simulink model "s_FPID_SOPDTUZ"  (R2022a)
settings: Solver=ode45  StartTime=0.0  StopTime=simT  MaxStep=Tsm  RelTol=rtol  AbsTol=atol
values from neighbouring files (symbols this model uses):
  beta = c0(5)+c1(5)*a+c2(5)*b+c3(5)*a*b+c4(5)*b^2+c5(5)*a*b^2+c6(5)*b^3    [PID_MoReRT.m]
  D1 = [T^2 2*T 1]    [Figure_08.m]    (also in PD1nR_2DOF_Qn.m; PD3nR_2DOF_Qn.m; PD5nR_2DOF_Qn.m; PD7nR_2DOF_Qn.m)
  di0 = 0    [Figure_03a_above.m]    (also in Figure_03b_middle.m; Figure_03c_below.m; Figure_04.m; Figure_05.m)
  di1 = 1    [Figure_03a_above.m]    (also in Figure_03b_middle.m; Figure_03c_below.m; Figure_04.m; Figure_05.m)
  do = 0    [Figure_03a_above.m]    (also in Figure_03b_middle.m; Figure_03c_below.m; Figure_04.m; Figure_05.m)
  do0 = 0    [Figure_03a_above.m]    (also in Figure_03b_middle.m; Figure_03c_below.m; Figure_04.m; Figure_05.m)
  dy = .1    (= 0.1)    [Figure_03a_above.m]    (also in Figure_03b_middle.m; Figure_03c_below.m; Figure_04.m = 0.05; Figure_05.m = 0.05)
  Kdy = 0    [Figure_03a_above.m]    (also in Figure_03b_middle.m; Figure_03c_below.m; Figure_04.m; Figure_05.m)
  Kp = kp/K    [PID_MoReRT.m]
  N1 = K*[-T0 1]    [Figure_08.m]    (also in PD1nR_2DOF_Qn.m; PD3nR_2DOF_Qn.m; PD5nR_2DOF_Qn.m; PD7nR_2DOF_Qn.m)
  TD = td*T    [PID_MoReRT.m]
  Tf = Te/n    (= 0.436)    [Figure_03a_above.m]    (also in Figure_03b_middle.m = 0.218; Figure_03c_below.m = 0.254333333333; Figure_04.m = Te/n; Figure_05.m = Te/n)
  ti = Ts    (= 0.001)    [Figure_03a_above.m]    (also in Figure_03b_middle.m; Figure_03c_below.m; Figure_04.m; Figure_05.m)
  Ti = taui*Td    [PD1nR_2DOF_Qn.m]    (also in PD1nR_NcPn.m; PD3nR_2DOF_Qn.m; PD3nR_NcPn.m; PD5nR_2DOF_Qn.m)
  to = Ts    (= 0.001)    [Figure_03a_above.m]    (also in Figure_03b_middle.m; Figure_03c_below.m; Figure_04.m; Figure_05.m)
  Ts = 0.001    [Figure_03a_above.m]    (also in Figure_03b_middle.m; Figure_03c_below.m; Figure_04.m; Figure_05.m)
  tw = Ts    (= 0.001)    [Figure_03a_above.m]    (also in Figure_03b_middle.m; Figure_03c_below.m; Figure_04.m; Figure_05.m)
  Umax = 10    [Figure_03a_above.m]    (also in Figure_03b_middle.m; Figure_03c_below.m; Figure_04.m; Figure_05.m)
  Umin = -10    [Figure_03a_above.m]    (also in Figure_03b_middle.m; Figure_03c_below.m; Figure_04.m; Figure_05.m)
  w0 = 0    [Figure_03a_above.m]    (also in Figure_03b_middle.m; Figure_03c_below.m; Figure_04.m; Figure_05.m)
  w1 = 0    [Figure_03a_above.m]    (also in Figure_03b_middle.m; Figure_03c_below.m; Figure_04.m; Figure_05.m)
settings Model: ExtModeTrigMode=oneshot  ExtModeArmWhenConnect=off  Creator=mhuba  LastModifiedBy=pbistak
settings SolverCC: AutoScaleAbsTol=off  AlgebraicLoopSolver=TrustRegion
settings DataIOCC: SaveFormat=Array  SignalLoggingSaveFormat=ModelDataLogs  ReturnWorkspaceOutputs=off  SignalLoggingName=sigsOut
settings OptimizationCC: BooleanDataType=off  ExpressionDepthLimit=2147483647  LifeSpan=inf
settings DebuggingCC: SaveWithParameterizedLinksMsg=none  UnderspecifiedInitializationDetection=Classic  MergeDetectMultiDrivingBlocksExec=none  SignalResolutionControl=TryResolveAllWithWarning  MultiTaskDSMMsg=warning  MultiTaskCondExecSysMsg=none  FcnCallInpInsideContextMsg=warning  UnconnectedInputMsg=warning  UnconnectedOutputMsg=warning  UnconnectedLineMsg=warning  StateNameClashWarn=warning  SFUnexpectedBacktrackingDiag=warning  SFNoUnconditionalDefaultTransitionDiag=warning  SFExecutionAtInitializationDiag=none  SFMachineParentedDataDiag=warning  ArithmeticOperatorsInVariantConditions=warning
settings HardwareCC: ProdBitPerPointer=32  ProdBitPerSizeT=32  ProdBitPerPtrDiffT=32  ProdLargestAtomicFloat=None  ProdIntDivRoundTo=Undefined  ProdEndianess=Unspecified  ProdWordSize=32  ProdHWDeviceType=32-bit Generic  TargetUnknown=on
settings ModelReferenceCC: PropagateSignalLabelsOutOfModel=off
settings SFSimCC: SimUseLocalCustomCode=off  CustomCodeUndefinedFunction=UseInterfaceOnly
settings RTWCC: TemplateMakefile=grt_vc.tmf  RTWUseLocalCustomCode=off
settings CodeAppCC: StateflowObjectComments=on
settings GRTTargetCC: TargetLangStandard=C89/C90 (ANSI)  CombineOutputUpdateFcns=off  GRTInterface=on
settings ConfigComp: CovMetricSettings=dw  CovSaveCumulativeToWorkspaceVar=on  CovSaveSingleToWorkspaceVar=on  CovExternalEMLEnable=off

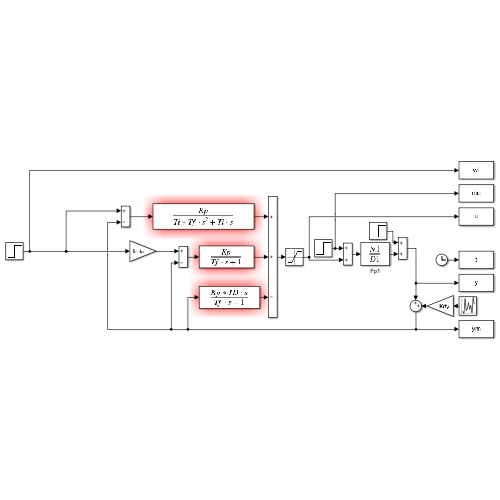
[thumbnail: Simulink's stored preview of the top-level diagram]
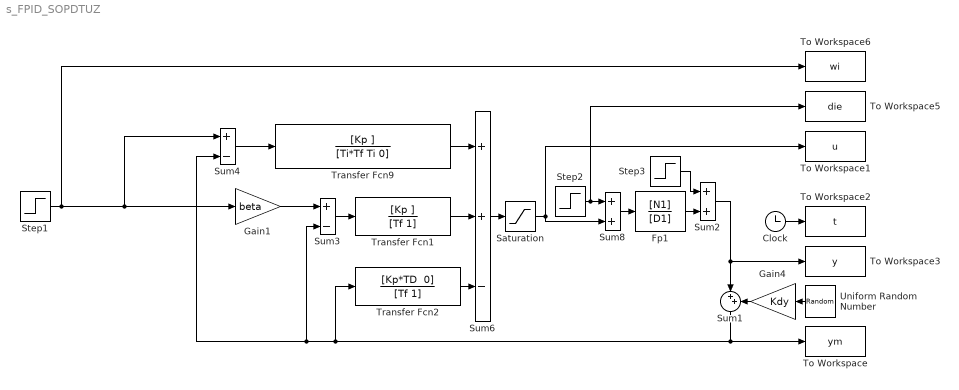
== system s_FPID_SOPDTUZ ==
  Clock : Clock
  Fp1 : TransferFcn  Numerator=[N1]  Denominator=[D1]
  Gain1 : Gain  Gain=beta  SaturateOnIntegerOverflow=on  OutDataTypeStr=Inherit: Same as input  ParamDataTypeStr=Inherit: Same as input
  Gain4 : Gain  Gain=Kdy  SaturateOnIntegerOverflow=on  OutDataTypeStr=Inherit: Same as input  ParamDataTypeStr=Inherit: Same as input
  Saturation : Saturate  UpperLimit=Umax  LowerLimit=Umin
  Step1 : Step  Time=tw  Before=w0  After=w1  SampleTime=Ts
  Step2 : Step  Time=ti  Before=di0  After=di1  SampleTime=Ts
  Step3 : Step  Time=to  Before=do0  After=do  SampleTime=Ts
  Sum1 : Sum  Inputs=|++  InputSameDT=on  SaturateOnIntegerOverflow=on  OutDataTypeStr=Inherit: Same as first input
  Sum2 : Sum  InputSameDT=on  SaturateOnIntegerOverflow=on  OutDataTypeStr=Inherit: Same as first input
  Sum3 : Sum  Inputs=+-  InputSameDT=on  SaturateOnIntegerOverflow=on  OutDataTypeStr=Inherit: Same as first input
  Sum4 : Sum  Inputs=+-  InputSameDT=on  SaturateOnIntegerOverflow=on  OutDataTypeStr=Inherit: Same as first input
  Sum6 : Sum  Inputs=++-  InputSameDT=on  SaturateOnIntegerOverflow=on  OutDataTypeStr=Inherit: Same as first input
  Sum8 : Sum  InputSameDT=on  SaturateOnIntegerOverflow=on  OutDataTypeStr=Inherit: Same as first input
  To Workspace : ToWorkspace  VariableName=ym  SampleTime=Ts
  To Workspace1 : ToWorkspace  VariableName=u  SampleTime=Ts
  To Workspace2 : ToWorkspace  VariableName=t  SampleTime=Ts
  To Workspace3 : ToWorkspace  VariableName=y  SampleTime=Ts
  To Workspace5 : ToWorkspace  VariableName=die  SampleTime=Ts
  To Workspace6 : ToWorkspace  VariableName=wi  SampleTime=Ts
  Transfer Fcn1 : TransferFcn  Numerator=[Kp ]  Denominator=[Tf 1]
  Transfer Fcn2 : TransferFcn  Numerator="[Kp*TD  0]"  Denominator=[Tf 1]
  Transfer Fcn9 : TransferFcn  Numerator=[Kp ]  Denominator=[Ti*Tf Ti 0]
  Uniform Random Number : UniformRandomNumber  Minimum=-dy  Maximum=dy  SampleTime=Ts
  wires:
  Step1/1 -> Sum4/1, Gain1/1, To Workspace6/1
  Sum8/1 -> Fp1/1
  Step2/1 -> Sum8/1, To Workspace5/1
  Clock/1 -> To Workspace2/1
  Sum2/1 -> Sum1/1, To Workspace3/1
  Uniform Random Number/1 -> Gain4/1
  Gain4/1 -> Sum1/2
  Step3/1 -> Sum2/1
  Fp1/1 -> Sum2/2
  Gain1/1 -> Sum3/1
  Sum1/1 -> To Workspace/1, Transfer Fcn2/1, Sum3/2, Sum4/2
  Transfer Fcn1/1 -> Sum6/2
  Transfer Fcn9/1 -> Sum6/1
  Sum6/1 -> Saturation/1
  Saturation/1 -> Sum8/2, To Workspace1/1
  Sum3/1 -> Transfer Fcn1/1
  Sum4/1 -> Transfer Fcn9/1
  Transfer Fcn2/1 -> Sum6/3
